simulink subsystem "Controller"  (R2023a)
settings: Solver=VariableStepAuto  StartTime=0.0  StopTime=10.0  RelTol=1e-3
model mask{kp=9, ki=7, Ts=0.01}
  mask prompts: kp "Proportional Gain"; ki "Integral Gain"; Ts "Sample Time"
undefined symbols (not defined in the file or in its folder): V
settings Model: Creator=MY PC  LastModifiedBy=MY PC

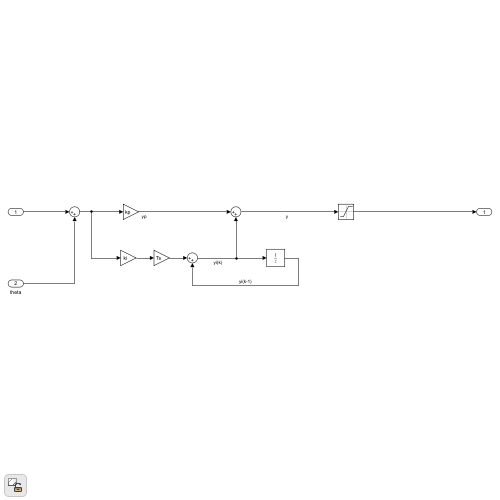
[thumbnail: Simulink's stored preview of the top-level diagram]
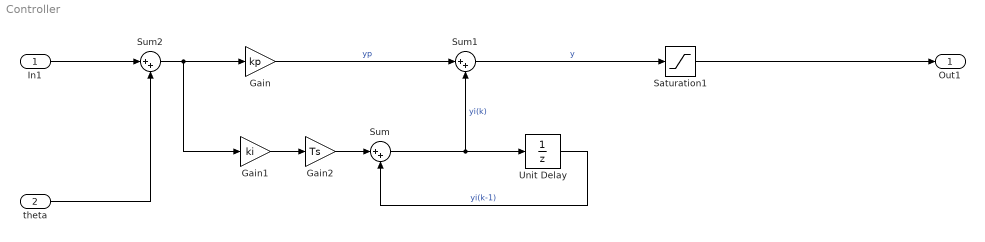
== system Controller ==
  In1 : Inport
  theta : Inport  Port=2
  Gain : Gain  Gain=kp
  Gain1 : Gain  Gain=ki
  Gain2 : Gain  Gain=Ts
  Saturation1 : Saturate  UpperLimit=V  LowerLimit=-V
  Sum : Sum  Inputs=|++
  Sum1 : Sum  Inputs=|++
  Sum2 : Sum  Inputs=|++
  Unit Delay : UnitDelay  SampleTime=Ts  HasFrameUpgradeWarning=on
  Out1 : Outport
  wires:
  Gain/1 -> Sum1/1  "yp"
  Sum/1 -> Unit Delay/1, Sum1/2  "yi(k)"
  Sum2/1 -> Gain/1, Gain1/1
  Gain1/1 -> Gain2/1
  Unit Delay/1 -> Sum/2  "yi(k-1)"
  Sum1/1 -> Saturation1/1  "y"
  Saturation1/1 -> Out1/1
  Gain2/1 -> Sum/1
  In1/1 -> Sum2/1
  theta/1 -> Sum2/2
